simulink model "r3r4calc"  (R2018b)
settings: Solver=VariableStepAuto  StartTime=0.0  StopTime=10.0  RelTol=1e-3
settings Model: Creator=Cole  LastModifiedBy=Cole

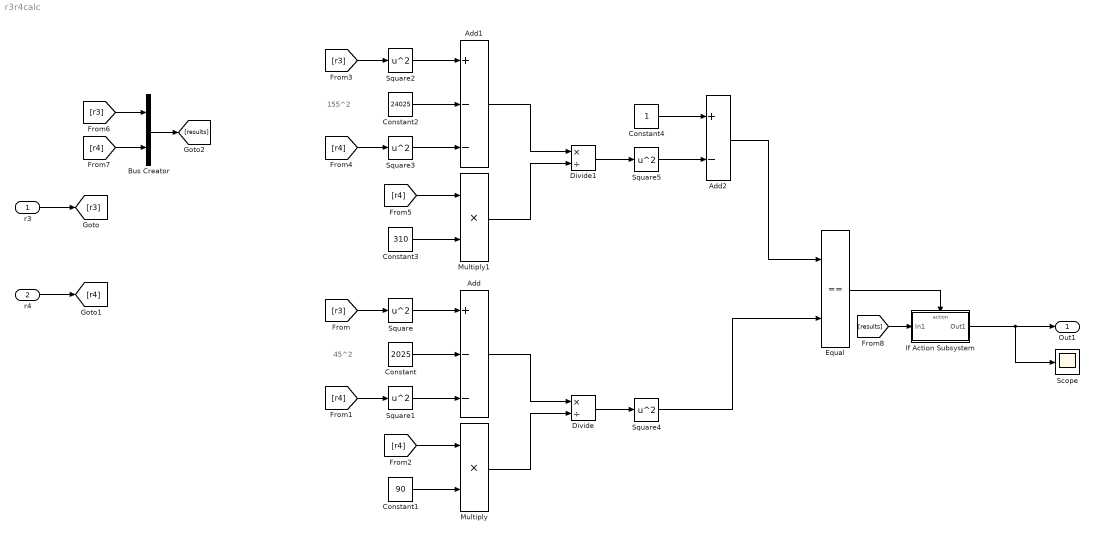
== system r3r4calc ==
  note: 45^2
  note: 155^2
  r3 : Inport
  r4 : Inport  Port=2
  Add : Sum  Inputs=+--
  Add1 : Sum  Inputs=+--
  Add2 : Sum  Inputs=+-
  Bus Creator : BusCreator  Inputs=2
  Constant : Constant  Value=2025
  Constant1 : Constant  Value=90
  Constant2 : Constant  Value=24025
  Constant3 : Constant  Value=310
  Constant4 : Constant
  Divide : Product  Inputs=*/
  Divide1 : Product  Inputs=*/
  Equal : RelationalOperator  Operator===  OutDataTypeStr=boolean  RndMeth=Simplest
  If Action Subsystem : Subsystem  TreatAsAtomicUnit=on
  Multiply : Product
  Multiply1 : Product
  Scope : Scope
  Square{,1..5} (6 alike) : Math  Operator=square  SaturateOnIntegerOverflow=on
  Out1 : Outport
  wires:
  Constant/1 -> Add/2
  Square/1 -> Add/1
  Square1/1 -> Add/3
  Constant1/1 -> Multiply/2
  Add/1 -> Divide/1
  Multiply/1 -> Divide/2
  r3/1 -> [r3]
  [r3] -> Square/1
  r4/1 -> [r4]
  [r4] -> Multiply/1
  [r4] -> Square1/1
  [r3] -> Square2/1
  Square2/1 -> Add1/1
  Add1/1 -> Divide1/1
  Multiply1/1 -> Divide1/2
  Square3/1 -> Add1/3
  Constant2/1 -> Add1/2
  [r4] -> Square3/1
  Constant3/1 -> Multiply1/2
  [r4] -> Multiply1/1
  Divide/1 -> Square4/1
  Divide1/1 -> Square5/1
  Square5/1 -> Add2/2
  Constant4/1 -> Add2/1
  Square4/1 -> Equal/2
  Add2/1 -> Equal/1
  Equal/1 -> If Action Subsystem/Action
  [r3] -> Bus Creator/1
  [r4] -> Bus Creator/2
  Bus Creator/1 -> [results]
  If Action Subsystem/1(Out1) -> Out1/1, Scope/1
  [results] -> If Action Subsystem/1(In1)

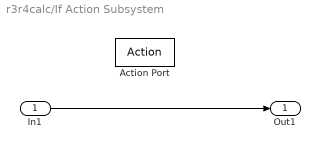
== system r3r4calc/If Action Subsystem ==
  In1 : Inport
  Action Port : ActionPort
  Out1 : Outport
  wires:
  In1/1 -> Out1/1
